simulink model "rotation"  (Simulink 7.0)
settings: Solver=ode45  SolverMode=SingleTasking  StartTime=0.0  StopTime=inf  RelTol=1e-3
values from neighbouring files (symbols this model uses):
  blk = 10    [rotation_init.m]
  col_delx_ws = ceil(col_delx*2^20)    [rotation_init.m]
  col_dely_ws = ceil(col_dely*2^20)    [rotation_init.m]
  fps = 1/(rows*(cols+3*blk))    [rotation_init.m]
  row_delx_ws = ceil(row_delx*2^20)*2    [rotation_init.m]
  row_dely_ws = ceil(row_dely*2^20)*2    [rotation_init.m]
  xstart_init_ws = ceil(xstart_init*2^20)    [rotation_init.m]
  ystart_init_ws = ceil(ystart_init*2^20)    [rotation_init.m]
undefined symbols (not defined in the file or in its folder): cols, rows
libraries: xbsIndex_r4 x273, dspsrcs4 x2, dspsigops x1, vipsrcs x1
(part 1 of 2)
settings Model: Creator=Neelamegam Subramani  LastModifiedBy=IC011758
settings DataIOCC: SaveOutput=off  SignalLogging=off  SaveTime=off

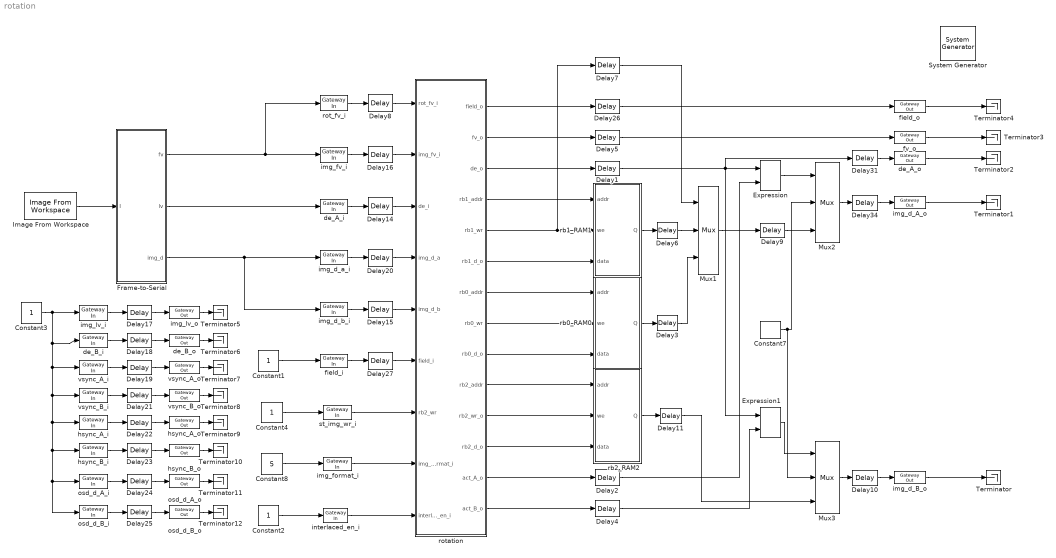
== system rotation ==
  " System Generator" : xbsIndex_r4/ System Generator  Tag=genX  SystemSampleTime=-1  xilinxfamily=spartan3adsp  part=xc3sd3400a  speed=-5  package=fg676  synthesis_tool=XST  clock_wrapper=Clock Enables  directory=./ngc_netlist  testbench=off  simulink_period=(1/fps)/ (rows*(cols+2*blk))  sysclk_period=(1/110e6)*1e9  dcm_input_clock_period=100  incr_netlist=off  trim_vbits=Everywhere in SubSystem  dbl_ovrd=According to Block Masks  core_generation=According to Block Masks  run_coregen=off  deprecated_control=off  eval_field=0  block_type=sysgen
      settings: block_version=8.2
  Constant{1..4} (4 alike) : Constant  OutDataType=sfix(16)  OutScaling=2^0
  Constant7 : xbsIndex_r4/Constant  arith_type=Unsigned  const=0  n_bits=10  bin_pt=0  explicit_period=on  period=(1/fps)/ (rows*(cols+2*blk))  equ=P=C  opselect=C  inp2=PCIN>>17  opr=+  inp1=P  carry=CIN  dbl_ovrd=off  block_type=constant
  Constant8 : Constant  Value=5  OutDataType=sfix(16)  OutScaling=2^0
  Delay1 : xbsIndex_r4/Delay  en=off  latency=5  dbl_ovrd=off  reg_retiming=off  block_type=delay
  Delay{3,6,8..10,14..16,20,27,31,34} (12 alike) : xbsIndex_r4/Delay  en=off  latency=1  dbl_ovrd=off  reg_retiming=off  block_type=delay
      Delay10 settings: infoedit="Delay line having  configurable length.<P><P>Hardware notes: A delay line is a chain, each link of which is an SRL16 followed by a flip-flop. If register retiming is enabled, the delay line is a chain of flip-flops."  xl_area=[0, 0, 0, 0, 0, 0, 0]  block_version=VER_STRING_GOES_HERE
      Delay3 settings: infoedit="Delay line having  configurable length.<P><P>Hardware notes: A delay line is a chain, each link of which is an SRL16 followed by a flip-flop. If register retiming is enabled, the delay line is a chain of flip-flops."  xl_area=[0, 0, 0, 0, 0, 0, 0]  block_version=VER_STRING_GOES_HERE
      Delay31 settings: infoedit="Delay line having  configurable length.<P><P>Hardware notes: A delay line is a chain, each link of which is an SRL16 followed by a flip-flop. If register retiming is enabled, the delay line is a chain of flip-flops."  xl_area=[0, 0, 0, 0, 0, 0, 0]  block_version=VER_STRING_GOES_HERE
      Delay34 settings: infoedit="Delay line having  configurable length.<P><P>Hardware notes: A delay line is a chain, each link of which is an SRL16 followed by a flip-flop. If register retiming is enabled, the delay line is a chain of flip-flops."  xl_area=[0, 0, 0, 0, 0, 0, 0]  block_version=VER_STRING_GOES_HERE
      Delay6 settings: infoedit="Delay line having  configurable length.<P><P>Hardware notes: A delay line is a chain, each link of which is an SRL16 followed by a flip-flop. If register retiming is enabled, the delay line is a chain of flip-flops."  xl_area=[0, 0, 0, 0, 0, 0, 0]  block_version=VER_STRING_GOES_HERE
  Delay11 : xbsIndex_r4/Delay  en=off  latency=2  dbl_ovrd=off  reg_retiming=off  block_type=delay
      settings: infoedit="Delay line having  configurable length.<P><P>Hardware notes: A delay line is a chain, each link of which is an SRL16 followed by a flip-flop. If register retiming is enabled, the delay line is a chain of flip-flops."  xl_area=[0, 0, 0, 0, 0, 0, 0]  block_version=VER_STRING_GOES_HERE
  Delay{17..19,21..25} (8 alike) : xbsIndex_r4/Delay  en=off  latency=15  dbl_ovrd=off  reg_retiming=off  block_type=delay
  Delay2 : xbsIndex_r4/Delay  en=off  latency=5  dbl_ovrd=off  reg_retiming=off  block_type=delay
      settings: infoedit="Delay line having  configurable length.<P><P>Hardware notes: A delay line is a chain, each link of which is an SRL16 followed by a flip-flop. If register retiming is enabled, the delay line is a chain of flip-flops."  xl_area=[0, 0, 0, 0, 0, 0, 0]  block_version=VER_STRING_GOES_HERE
  Delay26 : xbsIndex_r4/Delay  en=off  latency=6  dbl_ovrd=off  reg_retiming=off  block_type=delay
  Delay4 : xbsIndex_r4/Delay  en=off  latency=5  dbl_ovrd=off  reg_retiming=off  block_type=delay
      settings: infoedit="Delay line having  configurable length.<P><P>Hardware notes: A delay line is a chain, each link of which is an SRL16 followed by a flip-flop. If register retiming is enabled, the delay line is a chain of flip-flops."  xl_area=[0, 0, 0, 0, 0, 0, 0]  block_version=VER_STRING_GOES_HERE
  Delay5 : xbsIndex_r4/Delay  en=off  latency=6  dbl_ovrd=off  reg_retiming=off  block_type=delay
  Delay7 : xbsIndex_r4/Delay  en=off  latency=3  dbl_ovrd=off  reg_retiming=off  block_type=delay
      settings: infoedit="Delay line having  configurable length.<P><P>Hardware notes: A delay line is a chain, each link of which is an SRL16 followed by a flip-flop. If register retiming is enabled, the delay line is a chain of flip-flops."  xl_area=[0, 0, 0, 0, 0, 0, 0]  block_version=VER_STRING_GOES_HERE
  Expression : xbsIndex_r4/Expression  expression=a & b  align_bp=on  en=off  latency=0  precision=Full  arith_type=Unsigned  n_bits=16  bin_pt=0  dbl_ovrd=off  block_type=expr
      settings: block_version=10.1.3
  Expression1 : xbsIndex_r4/Expression  expression=a & b  align_bp=on  en=off  latency=0  precision=Full  arith_type=Unsigned  n_bits=16  bin_pt=0  dbl_ovrd=off  block_type=expr
      settings: block_version=10.1.3
  Frame-to-Serial : Subsystem
  Image From Workspace : vipsrcs/Image From Workspace  Tag=vipblks_nd  SystemSampleTime=-1  ImageValue=in  Ts=1/fps  imagePorts=One multidimensional signal  ImageDataType=double  Signed=on  WordLength=16  sdImageDataType=sfix(16)  FractionLengthMode=User-defined  FractionLength=15  OutPortLabels=R|G|B
      link override Constant1: Value=ImageValue
  Mux1 : xbsIndex_r4/Mux  inputs=2  en=off  latency=0  precision=Full  arith_type=Unsigned  n_bits=16  bin_pt=14  quantization=Truncate  overflow=Wrap  dbl_ovrd=off  block_type=mux
  Mux2 : xbsIndex_r4/Mux  inputs=2  en=off  latency=0  precision=Full  arith_type=Unsigned  n_bits=16  bin_pt=14  quantization=Truncate  overflow=Wrap  dbl_ovrd=off  block_type=mux
  Mux3 : xbsIndex_r4/Mux  inputs=2  en=off  latency=0  precision=Full  arith_type=Unsigned  n_bits=16  bin_pt=14  quantization=Truncate  overflow=Wrap  dbl_ovrd=off  block_type=mux
  Terminator{,1..12} (13 alike) : Terminator
  de_A_i : xbsIndex_r4/Gateway In  arith_type=Boolean  n_bits=10  bin_pt=0  quantization=Truncate  overflow=Wrap  period=(1/fps)/ (rows*(cols+2*blk))  dbl_ovrd=off  timing_constraint=None  locs_specified=off  LOCs={}  block_type=gatewayin
      settings: infoedit="Gateway in block.  Converts inputs of type Simulink integer, double and fixed point to  Xilinx fixed point type.<P><P>Hardware notes:  In hardware these blocks become top level input ports."  block_version=10.1.3
  de_A_o : xbsIndex_r4/Gateway Out  hdl_port=on  timing_constraint=None  locs_specified=off  LOCs={'AC11'}  block_type=gatewayout
      settings: infoedit="Gateway out block.  Converts Xilinx fixed point inputs into ouputs of type Simulink integer, double, or fixed point.<P><P>Hardware notes:  In hardware these blocks become top level output ports or are discarded, depending on how they are configured."  block_version=10.1.3
  de_B_i : xbsIndex_r4/Gateway In  arith_type=Boolean  n_bits=10  bin_pt=0  quantization=Truncate  overflow=Wrap  period=(1/fps)/ (rows*(cols+2*blk))  dbl_ovrd=off  timing_constraint=None  locs_specified=off  LOCs={}  block_type=gatewayin
      settings: infoedit="Gateway in block.  Converts inputs of type Simulink integer, double and fixed point to  Xilinx fixed point type.<P><P>Hardware notes:  In hardware these blocks become top level input ports."  block_version=10.1.3
  de_B_o : xbsIndex_r4/Gateway Out  hdl_port=on  timing_constraint=None  locs_specified=off  LOCs={}  block_type=gatewayout
      settings: infoedit="Gateway out block.  Converts Xilinx fixed point inputs into ouputs of type Simulink integer, double, or fixed point.<P><P>Hardware notes:  In hardware these blocks become top level output ports or are discarded, depending on how they are configured."  block_version=10.1.3
  field_i : xbsIndex_r4/Gateway In  arith_type=Boolean  n_bits=16  bin_pt=14  quantization="Round  (unbiased: +/- Inf)"  overflow=Saturate  period=(1/fps)/ (rows*(cols+2*blk))  dbl_ovrd=off  timing_constraint=None  locs_specified=off  LOCs={}  block_type=gatewayin
      settings: infoedit="Gateway in block.  Converts inputs of type Simulink integer, double and fixed point to  Xilinx fixed point type.<P><P>Hardware notes:  In hardware these blocks become top level input ports."  block_version=10.1.3
  field_o : xbsIndex_r4/Gateway Out  hdl_port=on  timing_constraint=None  locs_specified=off  LOCs={}  block_type=gatewayout
      settings: infoedit="Gateway out block.  Converts Xilinx fixed point inputs into ouputs of type Simulink integer, double, or fixed point.<P><P>Hardware notes:  In hardware these blocks become top level output ports or are discarded, depending on how they are configured."  block_version=10.1.3
  fv_o : xbsIndex_r4/Gateway Out  hdl_port=on  timing_constraint=None  locs_specified=off  LOCs={'AD11'}  block_type=gatewayout
      settings: infoedit="Gateway out block.  Converts Xilinx fixed point inputs into ouputs of type Simulink integer, double, or fixed point.<P><P>Hardware notes:  In hardware these blocks become top level output ports or are discarded, depending on how they are configured."  block_version=10.1.3
  hsync_A_i : xbsIndex_r4/Gateway In  arith_type=Boolean  n_bits=10  bin_pt=0  quantization=Truncate  overflow=Wrap  period=(1/fps)/ (rows*(cols+2*blk))  dbl_ovrd=off  timing_constraint=None  locs_specified=off  LOCs={}  block_type=gatewayin
      settings: infoedit="Gateway in block.  Converts inputs of type Simulink integer, double and fixed point to  Xilinx fixed point type.<P><P>Hardware notes:  In hardware these blocks become top level input ports."  block_version=10.1.3
  hsync_A_o : xbsIndex_r4/Gateway Out  hdl_port=on  timing_constraint=None  locs_specified=off  LOCs={}  block_type=gatewayout
      settings: infoedit="Gateway out block.  Converts Xilinx fixed point inputs into ouputs of type Simulink integer, double, or fixed point.<P><P>Hardware notes:  In hardware these blocks become top level output ports or are discarded, depending on how they are configured."  block_version=10.1.3
  hsync_B_i : xbsIndex_r4/Gateway In  arith_type=Boolean  n_bits=10  bin_pt=0  quantization=Truncate  overflow=Wrap  period=(1/fps)/ (rows*(cols+2*blk))  dbl_ovrd=off  timing_constraint=None  locs_specified=off  LOCs={}  block_type=gatewayin
      settings: infoedit="Gateway in block.  Converts inputs of type Simulink integer, double and fixed point to  Xilinx fixed point type.<P><P>Hardware notes:  In hardware these blocks become top level input ports."  block_version=10.1.3
  hsync_B_o : xbsIndex_r4/Gateway Out  hdl_port=on  timing_constraint=None  locs_specified=off  LOCs={}  block_type=gatewayout
      settings: infoedit="Gateway out block.  Converts Xilinx fixed point inputs into ouputs of type Simulink integer, double, or fixed point.<P><P>Hardware notes:  In hardware these blocks become top level output ports or are discarded, depending on how they are configured."  block_version=10.1.3
  img_d_A_o : xbsIndex_r4/Gateway Out  hdl_port=on  timing_constraint=None  locs_specified=off  LOCs={}  block_type=gatewayout
      settings: infoedit="Gateway out block.  Converts Xilinx fixed point inputs into ouputs of type Simulink integer, double, or fixed point.<P><P>Hardware notes:  In hardware these blocks become top level output ports or are discarded, depending on how they are configured."  block_version=10.1.3
  img_d_B_o : xbsIndex_r4/Gateway Out  hdl_port=on  timing_constraint=None  locs_specified=off  LOCs={}  block_type=gatewayout
      settings: infoedit="Gateway out block.  Converts Xilinx fixed point inputs into ouputs of type Simulink integer, double, or fixed point.<P><P>Hardware notes:  In hardware these blocks become top level output ports or are discarded, depending on how they are configured."  block_version=10.1.3
  img_d_a_i : xbsIndex_r4/Gateway In  arith_type=Unsigned  n_bits=10  bin_pt=0  quantization=Truncate  overflow=Wrap  period=(1/fps)/ (rows*(cols+2*blk))  dbl_ovrd=off  timing_constraint=None  locs_specified=off  LOCs={}  block_type=gatewayin
      settings: infoedit="Gateway in block.  Converts inputs of type Simulink integer, double and fixed point to  Xilinx fixed point type.<P><P>Hardware notes:  In hardware these blocks become top level input ports."  block_version=10.1.3
  img_d_b_i : xbsIndex_r4/Gateway In  arith_type=Unsigned  n_bits=10  bin_pt=0  quantization=Truncate  overflow=Wrap  period=(1/fps)/ (rows*(cols+2*blk))  dbl_ovrd=off  timing_constraint=None  locs_specified=off  LOCs={}  block_type=gatewayin
      settings: infoedit="Gateway in block.  Converts inputs of type Simulink integer, double and fixed point to  Xilinx fixed point type.<P><P>Hardware notes:  In hardware these blocks become top level input ports."  block_version=10.1.3
  img_format_i : xbsIndex_r4/Gateway In  arith_type=Unsigned  n_bits=3  bin_pt=0  quantization=Truncate  overflow=Wrap  period=(1/fps)/ (rows*(cols+2*blk))  dbl_ovrd=off  timing_constraint=None  locs_specified=off  LOCs={}  block_type=gatewayin
      settings: infoedit="Gateway in block.  Converts inputs of type Simulink integer, double and fixed point to  Xilinx fixed point type.<P><P>Hardware notes:  In hardware these blocks become top level input ports."  block_version=10.1.3
  img_fv_i : xbsIndex_r4/Gateway In  arith_type=Boolean  n_bits=16  bin_pt=14  quantization="Round  (unbiased: +/- Inf)"  overflow=Saturate  period=(1/fps)/ (rows*(cols+2*blk))  dbl_ovrd=off  timing_constraint=None  locs_specified=off  LOCs={}  block_type=gatewayin
      settings: infoedit="Gateway in block.  Converts inputs of type Simulink integer, double and fixed point to  Xilinx fixed point type.<P><P>Hardware notes:  In hardware these blocks become top level input ports."  block_version=10.1.3
  img_lv_i : xbsIndex_r4/Gateway In  arith_type=Boolean  n_bits=16  bin_pt=14  quantization="Round  (unbiased: +/- Inf)"  overflow=Saturate  period=(1/fps)/ (rows*(cols+2*blk))  dbl_ovrd=off  timing_constraint=None  locs_specified=off  LOCs={}  block_type=gatewayin
      settings: infoedit="Gateway in block.  Converts inputs of type Simulink integer, double and fixed point to  Xilinx fixed point type.<P><P>Hardware notes:  In hardware these blocks become top level input ports."  block_version=10.1.3
  img_lv_o : xbsIndex_r4/Gateway Out  hdl_port=on  timing_constraint=None  locs_specified=off  LOCs={}  block_type=gatewayout
      settings: infoedit="Gateway out block.  Converts Xilinx fixed point inputs into ouputs of type Simulink integer, double, or fixed point.<P><P>Hardware notes:  In hardware these blocks become top level output ports or are discarded, depending on how they are configured."  block_version=10.1.3
  interlaced_en_i : xbsIndex_r4/Gateway In  arith_type=Boolean  n_bits=16  bin_pt=14  quantization="Round  (unbiased: +/- Inf)"  overflow=Saturate  period=(1/fps)/ (rows*(cols+2*blk))  dbl_ovrd=off  timing_constraint=None  locs_specified=off  LOCs={}  block_type=gatewayin
      settings: infoedit="Gateway in block.  Converts inputs of type Simulink integer, double and fixed point to  Xilinx fixed point type.<P><P>Hardware notes:  In hardware these blocks become top level input ports."  block_version=10.1.3
  osd_d_A_i : xbsIndex_r4/Gateway In  arith_type=Unsigned  n_bits=2  bin_pt=0  quantization=Truncate  overflow=Wrap  period=(1/fps)/ (rows*(cols+2*blk))  dbl_ovrd=off  timing_constraint=None  locs_specified=off  LOCs={}  block_type=gatewayin
      settings: infoedit="Gateway in block.  Converts inputs of type Simulink integer, double and fixed point to  Xilinx fixed point type.<P><P>Hardware notes:  In hardware these blocks become top level input ports."  block_version=10.1.3
  osd_d_A_o : xbsIndex_r4/Gateway Out  hdl_port=on  timing_constraint=None  locs_specified=off  LOCs={}  block_type=gatewayout
      settings: infoedit="Gateway out block.  Converts Xilinx fixed point inputs into ouputs of type Simulink integer, double, or fixed point.<P><P>Hardware notes:  In hardware these blocks become top level output ports or are discarded, depending on how they are configured."  block_version=10.1.3
  osd_d_B_i : xbsIndex_r4/Gateway In  arith_type=Unsigned  n_bits=2  bin_pt=0  quantization=Truncate  overflow=Wrap  period=(1/fps)/ (rows*(cols+2*blk))  dbl_ovrd=off  timing_constraint=None  locs_specified=off  LOCs={}  block_type=gatewayin
      settings: infoedit="Gateway in block.  Converts inputs of type Simulink integer, double and fixed point to  Xilinx fixed point type.<P><P>Hardware notes:  In hardware these blocks become top level input ports."  block_version=10.1.3
  osd_d_B_o : xbsIndex_r4/Gateway Out  hdl_port=on  timing_constraint=None  locs_specified=off  LOCs={}  block_type=gatewayout
      settings: infoedit="Gateway out block.  Converts Xilinx fixed point inputs into ouputs of type Simulink integer, double, or fixed point.<P><P>Hardware notes:  In hardware these blocks become top level output ports or are discarded, depending on how they are configured."  block_version=10.1.3
  rb0_RAM0 : Subsystem  AncestorBlock=XtremeDSPKit_r4/External RAM  mask(XtremeDSP Kit External Memory){zbt_data_read_arith_type=Unsigned, zbt_data_width=16, zbt_data_bin_pt=0}
      mask prompts: zbt_data_read_arith_type "Output Data Type"; zbt_data_width "Data Width"; zbt_data_bin_pt "Data Binary Point (from 0 to 16)"
      mask help: 256K x 16 External Memory
      mask init:
      | i = imread('xtreme.jpg');
      mask Help: eval('');xlDoc('-book','sysgen','-topic','XtremeDSP_External_RAM');
      mask StyleString: popup(Unsigned|Signed  (2's comp)),edit,edit
      mask Display:
      | image(i);
      | port_label ('input', 1, 'addr');
      | port_label ('input', 2, 'we');
      | port_label ('input', 3, 'data');
  rb1_RAM1 : Subsystem  AncestorBlock=XtremeDSPKit_r4/External RAM  mask(XtremeDSP Kit External Memory){zbt_data_read_arith_type=Unsigned, zbt_data_width=16, zbt_data_bin_pt=0}
      mask prompts: zbt_data_read_arith_type "Output Data Type"; zbt_data_width "Data Width"; zbt_data_bin_pt "Data Binary Point (from 0 to 16)"
      mask help: 256K x 16 External Memory
      mask init:
      | i = imread('xtreme.jpg');
      mask Help: eval('');xlDoc('-book','sysgen','-topic','XtremeDSP_External_RAM');
      mask StyleString: popup(Unsigned|Signed  (2's comp)),edit,edit
      mask Display:
      | image(i);
      | port_label ('input', 1, 'addr');
      | port_label ('input', 2, 'we');
      | port_label ('input', 3, 'data');
  rb2_RAM2 : Subsystem  AncestorBlock=XtremeDSPKit_r4/External RAM  mask(XtremeDSP Kit External Memory){zbt_data_read_arith_type=Unsigned, zbt_data_width=16, zbt_data_bin_pt=0}
      mask prompts: zbt_data_read_arith_type "Output Data Type"; zbt_data_width "Data Width"; zbt_data_bin_pt "Data Binary Point (from 0 to 16)"
      mask help: 256K x 16 External Memory
      mask init:
      | i = imread('xtreme.jpg');
      mask Help: eval('');xlDoc('-book','sysgen','-topic','XtremeDSP_External_RAM');
      mask StyleString: popup(Unsigned|Signed  (2's comp)),edit,edit
      mask Display:
      | image(i);
      | port_label ('input', 1, 'addr');
      | port_label ('input', 2, 'we');
      | port_label ('input', 3, 'data');
  rot_fv_i : xbsIndex_r4/Gateway In  arith_type=Boolean  n_bits=16  bin_pt=14  quantization="Round  (unbiased: +/- Inf)"  overflow=Saturate  period=(1/fps)/ (rows*(cols+2*blk))  dbl_ovrd=off  timing_constraint=None  locs_specified=off  LOCs={}  block_type=gatewayin
      settings: infoedit="Gateway in block.  Converts inputs of type Simulink integer, double and fixed point to  Xilinx fixed point type.<P><P>Hardware notes:  In hardware these blocks become top level input ports."  block_version=10.1.3
  rotation : Subsystem
  st_img_wr_i : xbsIndex_r4/Gateway In  arith_type=Boolean  n_bits=10  bin_pt=0  quantization=Truncate  overflow=Wrap  period=(1/fps)/ (rows*(cols+2*blk))  dbl_ovrd=off  timing_constraint=None  locs_specified=off  LOCs={}  block_type=gatewayin
      settings: infoedit="Gateway in block.  Converts inputs of type Simulink integer, double and fixed point to  Xilinx fixed point type.<P><P>Hardware notes:  In hardware these blocks become top level input ports."  block_version=10.1.3
  vsync_A_i : xbsIndex_r4/Gateway In  arith_type=Boolean  n_bits=10  bin_pt=0  quantization=Truncate  overflow=Wrap  period=(1/fps)/ (rows*(cols+2*blk))  dbl_ovrd=off  timing_constraint=None  locs_specified=off  LOCs={}  block_type=gatewayin
      settings: infoedit="Gateway in block.  Converts inputs of type Simulink integer, double and fixed point to  Xilinx fixed point type.<P><P>Hardware notes:  In hardware these blocks become top level input ports."  block_version=10.1.3
  vsync_A_o : xbsIndex_r4/Gateway Out  hdl_port=on  timing_constraint=None  locs_specified=off  LOCs={}  block_type=gatewayout
      settings: infoedit="Gateway out block.  Converts Xilinx fixed point inputs into ouputs of type Simulink integer, double, or fixed point.<P><P>Hardware notes:  In hardware these blocks become top level output ports or are discarded, depending on how they are configured."  block_version=10.1.3
  vsync_B_i : xbsIndex_r4/Gateway In  arith_type=Boolean  n_bits=10  bin_pt=0  quantization=Truncate  overflow=Wrap  period=(1/fps)/ (rows*(cols+2*blk))  dbl_ovrd=off  timing_constraint=None  locs_specified=off  LOCs={}  block_type=gatewayin
      settings: infoedit="Gateway in block.  Converts inputs of type Simulink integer, double and fixed point to  Xilinx fixed point type.<P><P>Hardware notes:  In hardware these blocks become top level input ports."  block_version=10.1.3
  vsync_B_o : xbsIndex_r4/Gateway Out  hdl_port=on  timing_constraint=None  locs_specified=off  LOCs={}  block_type=gatewayout
      settings: infoedit="Gateway out block.  Converts Xilinx fixed point inputs into ouputs of type Simulink integer, double, or fixed point.<P><P>Hardware notes:  In hardware these blocks become top level output ports or are discarded, depending on how they are configured."  block_version=10.1.3
  wires:
  Image From Workspace/1 -> Frame-to-Serial/1(I)
  rb1_RAM1/1(Q) -> Delay6/1
  rb0_RAM0/1(Q) -> Delay3/1
  Delay6/1 -> Mux1/2
  Delay3/1 -> Mux1/3
  Delay7/1 -> Mux1/1
  Mux1/1 -> Delay9/1
  rb2_RAM2/1(Q) -> Delay11/1
  img_d_B_o/1 -> Terminator/1
  img_d_a_i/1 -> Delay20/1
  Frame-to-Serial/2(lv) -> de_A_i/1
  Frame-to-Serial/3(img_d) -> img_d_a_i/1, img_d_b_i/1
  de_A_i/1 -> Delay14/1
  img_fv_i/1 -> Delay16/1
  Constant1/1 -> field_i/1
  img_d_b_i/1 -> Delay15/1
  field_i/1 -> Delay27/1
  Delay17/1 -> img_lv_o/1
  de_B_i/1 -> Delay18/1
  Delay18/1 -> de_B_o/1
  vsync_A_i/1 -> Delay19/1
  Delay19/1 -> vsync_A_o/1
  vsync_B_i/1 -> Delay21/1
  Delay21/1 -> vsync_B_o/1
  hsync_A_i/1 -> Delay22/1
  Delay22/1 -> hsync_A_o/1
  hsync_B_i/1 -> Delay23/1
  Delay23/1 -> hsync_B_o/1
  osd_d_A_i/1 -> Delay24/1
  Delay24/1 -> osd_d_A_o/1
  osd_d_B_i/1 -> Delay25/1
  Delay25/1 -> osd_d_B_o/1
  Constant3/1 -> osd_d_B_i/1, osd_d_A_i/1, hsync_B_i/1, hsync_A_i/1, vsync_B_i/1, vsync_A_i/1, de_B_i/1, img_lv_i/1
  img_lv_i/1 -> Delay17/1
  Frame-to-Serial/1(fv) -> img_fv_i/1, rot_fv_i/1
  rotation/12(rb2_d_o) -> rb2_RAM2/3(data)
  rotation/11(rb2_wr_o) -> rb2_RAM2/2(we)
  rotation/10(rb2_addr) -> rb2_RAM2/1(addr)
  rotation/9(rb0_d_o) -> rb0_RAM0/3(data)
  rotation/8(rb0_wr) -> rb0_RAM0/2(we)
  rotation/7(rb0_addr) -> rb0_RAM0/1(addr)
  rotation/6(rb1_d_o) -> rb1_RAM1/3(data)
  rotation/5(rb1_wr) -> Delay7/1, rb1_RAM1/2(we)
  rotation/4(rb1_addr) -> rb1_RAM1/1(addr)
  img_d_A_o/1 -> Terminator1/1
  Delay14/1 -> rotation/3(de_i)
  Delay20/1 -> rotation/4(img_d_a)
  Delay15/1 -> rotation/5(img_d_b)
  Delay27/1 -> rotation/6(field_i)
  Constant4/1 -> st_img_wr_i/1
  rotation/1(field_o) -> Delay26/1
  de_A_o/1 -> Terminator2/1
  fv_o/1 -> Terminator3/1
  field_o/1 -> Terminator4/1
  img_lv_o/1 -> Terminator5/1
  de_B_o/1 -> Terminator6/1
  vsync_A_o/1 -> Terminator7/1
  vsync_B_o/1 -> Terminator8/1
  hsync_A_o/1 -> Terminator9/1
  hsync_B_o/1 -> Terminator10/1
  osd_d_A_o/1 -> Terminator11/1
  osd_d_B_o/1 -> Terminator12/1
  Delay9/1 -> Mux2/3
  Mux2/1 -> Delay34/1
  Constant7/1 -> Mux2/2, Mux3/2
  Delay31/1 -> de_A_o/1
  Delay34/1 -> img_d_A_o/1
  img_format_i/1 -> rotation/8(img_format_i)
  Constant8/1 -> img_format_i/1
  Delay1/1 -> Delay31/1, Expression/1, Expression1/1
  rotation/3(de_o) -> Delay1/1
  Delay5/1 -> fv_o/1
  rotation/2(fv_o) -> Delay5/1
  Delay26/1 -> field_o/1
  st_img_wr_i/1 -> rotation/7(rb2_wr)
  rotation/13(act_A_o) -> Delay2/1
  rotation/14(act_B_o) -> Delay4/1
  Delay2/1 -> Expression/2
  Expression/1 -> Mux2/1
  Delay4/1 -> Expression1/2
  Expression1/1 -> Mux3/1
  Delay11/1 -> Mux3/3
  Mux3/1 -> Delay10/1
  Delay10/1 -> img_d_B_o/1
  rot_fv_i/1 -> Delay8/1
  Delay8/1 -> rotation/1(rot_fv_i)
  Delay16/1 -> rotation/2(img_fv_i)
  Constant2/1 -> interlaced_en_i/1
  interlaced_en_i/1 -> rotation/9(interlaced_en_i)

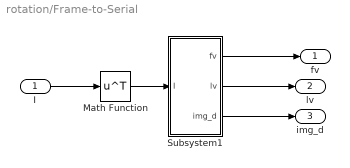
== system rotation/Frame-to-Serial ==
  I : Inport  OutDataType=sfix(16)  OutScaling=2^0
  Math Function : Math  Operator=transpose  SampleTime=(1/fps)  OutDataType=sfix(16)  OutScaling=2^0  SaturateOnIntegerOverflow=on
  Subsystem1 : Subsystem
  fv : Outport  OutDataType=sfix(16)  OutScaling=2^0
  lv : Outport  Port=2  OutDataType=sfix(16)  OutScaling=2^0
  img_d : Outport  Port=3  OutDataType=sfix(16)  OutScaling=2^0
  wires:
  I/1 -> Math Function/1
  Math Function/1 -> Subsystem1/1(I)
  Subsystem1/1(fv) -> fv/1
  Subsystem1/2(lv) -> lv/1
  Subsystem1/3(img_d) -> img_d/1

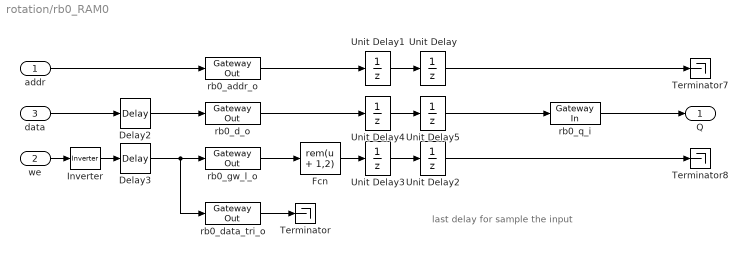
== system rotation/rb0_RAM0 ==
  note: last delay for sample the input
  addr : Inport  OutDataType=sfix(16)  OutScaling=2^0
  we : Inport  Port=2  OutDataType=sfix(16)  OutScaling=2^0
  data : Inport  Port=3  OutDataType=sfix(16)  OutScaling=2^0
  Delay2 : xbsIndex_r4/Delay  en=off  latency=1  dbl_ovrd=off  reg_retiming=off  block_type=delay
      settings: infoedit="Delay line having  configurable length.<P><P>Hardware notes: A delay line is a chain, each link of which is an SRL16 followed by a flip-flop. If register retiming is enabled, the delay line is a chain of flip-flops."  xl_area=[0, 0, 0, 0, 0, 0, 0]  block_version=VER_STRING_GOES_HERE
  Delay3 : xbsIndex_r4/Delay  en=off  latency=1  dbl_ovrd=off  reg_retiming=off  block_type=delay
      settings: infoedit="Delay line having  configurable length.<P><P>Hardware notes: A delay line is a chain, each link of which is an SRL16 followed by a flip-flop. If register retiming is enabled, the delay line is a chain of flip-flops."  xl_area=[0, 0, 0, 0, 0, 0, 0]  block_version=VER_STRING_GOES_HERE
  Fcn : Fcn  Expr=rem(u + 1,2)  SampleTime=(1/fps)/ (rows*(cols+2*blk))
  Inverter : xbsIndex_r4/Inverter  en=off  latency=0  dbl_ovrd=off  block_type=inv
      settings: xl_area=[0, 0, 0, 0, 0, 0, 0]  block_version=VER_STRING_GOES_HERE
  Terminator : Terminator
  Terminator7 : Terminator
  Terminator8 : Terminator
  Unit Delay{,1..5} (6 alike) : UnitDelay  SampleTime=(1/fps)/ (rows*(cols+2*blk))
  rb0_addr_o : xbsIndex_r4/Gateway Out  hdl_port=on  timing_constraint="Data Rate;  Set 'FAST' Attribute"  locs_specified=off  LOCs={'U1','U2','K6','L7','M10','M9','V2','V1','U4','T5','K3','K2','J5','J4','K5','K4','L4','L3'}  block_type=gatewayout
      settings: infoedit="Gateway out block.  Converts Xilinx fixed point inputs into ouputs of type Simulink integer, double, or fixed point.<P><P>Hardware notes:  In hardware these blocks become top level output ports or are discarded, depending on how they are configured."  xl_area=[0, 0, 0, 0, 0, 0, 0]  sginterface={'Nallatech'=>{'xdspkit'=>{'non_memory_mapped_port'=>'zbt_addr'}},'Xilinx'=>{'jtaghwcosim'=>{'non_memory_mapped_port'=>'zbt_addr'},'xdspkit'=>{'non_memory_mapped_port'=>'zbt_addr'}}}  block_version=VER_STRING_GOES_HERE
  rb0_d_o : xbsIndex_r4/Gateway Out  hdl_port=on  timing_constraint=None  locs_specified=off  LOCs={'B21','B22','A22','B23','B19','C19','A20','A21','A23','B24','A24','A25','E18','D18','C18','B18'}  block_type=gatewayout
      settings: infoedit="Gateway out block.  Converts Xilinx fixed point inputs into ouputs of type Simulink integer, double, or fixed point.<P><P>Hardware notes:  In hardware these blocks become top level output ports or are discarded, depending on how they are configured."  xl_area=[0, 0, 0, 0, 0, 0, 0]  sginterface={'Nallatech'=>{'xdspkit'=>{'non_memory_mapped_port'=>'zbt_data'}},'Xilinx'=>{'jtaghwcosim'=>{'non_memory_mapped_port'=>'zbt_data'},'xdspkit'=>{'non_memory_mapped_port'=>'zbt_data'}}}  block_version=VER_STRING_GOES_HERE
  rb0_data_tri_o : xbsIndex_r4/Gateway Out  hdl_port=on  timing_constraint=None  locs_specified=off  LOCs={}  block_type=gatewayout
      settings: infoedit="Gateway out block.  Converts Xilinx fixed point inputs into ouputs of type Simulink integer, double, or fixed point.<P><P>Hardware notes:  In hardware these blocks become top level output ports or are discarded, depending on how they are configured."  xl_area=[0, 0, 0, 0, 0, 0, 0]  sginterface={'Nallatech'=>{'xdspkit'=>{'non_memory_mapped_port'=>'zbt_data_tri'}},'Xilinx'=>{'jtaghwcosim'=>{'non_memory_mapped_port'=>'zbt_data_tri'},'xdspkit'=>{'non_memory_mapped_port'=>'zbt_data_tri'}}}  block_version=VER_STRING_GOES_HERE
  rb0_gw_l_o : xbsIndex_r4/Gateway Out  hdl_port=on  timing_constraint=None  locs_specified=off  LOCs={'A14'}  block_type=gatewayout
      settings: infoedit="Gateway out block.  Converts Xilinx fixed point inputs into ouputs of type Simulink integer, double, or fixed point.<P><P>Hardware notes:  In hardware these blocks become top level output ports or are discarded, depending on how they are configured."  xl_area=[0, 0, 0, 0, 0, 0, 0]  sginterface={'Nallatech'=>{'xdspkit'=>{'non_memory_mapped_port'=>'zbt_rd_wr'}},'Xilinx'=>{'jtaghwcosim'=>{'non_memory_mapped_port'=>'zbt_rd_wr'},'xdspkit'=>{'non_memory_mapped_port'=>'zbt_rd_wr'}}}  block_version=VER_STRING_GOES_HERE
  rb0_q_i : xbsIndex_r4/Gateway In  arith_type=Unsigned  n_bits=10  bin_pt=0  quantization=Truncate  overflow=Wrap  period=(1/fps)/ (rows*(cols+2*blk))  dbl_ovrd=off  timing_constraint=None  locs_specified=off  LOCs={}  block_type=gatewayin
      settings: infoedit="Gateway in block.  Converts inputs of type Simulink integer, double and fixed point to  Xilinx fixed point type.<P><P>Hardware notes:  In hardware these blocks become top level input ports."  xl_area=[0, 0, 0, 0, 0, 0, 0]  sginterface={'Nallatech'=>{'xdspkit'=>{'non_memory_mapped_port'=>'zbt_data_read'}},'Xilinx'=>{'jtaghwcosim'=>{'non_memory_mapped_port'=>'zbt_data_read'},'xdspkit'=>{'non_memory_mapped_port'=>'zbt_data_read'}}}  block_version=VER_STRING_GOES_HERE
  Q : Outport  OutDataType=sfix(16)  OutScaling=2^0
  wires:
  Inverter/1 -> Delay3/1
  Fcn/1 -> Unit Delay3/1
  rb0_gw_l_o/1 -> Fcn/1
  data/1 -> Delay2/1
  rb0_data_tri_o/1 -> Terminator/1
  addr/1 -> rb0_addr_o/1
  we/1 -> Inverter/1
  Unit Delay1/1 -> Unit Delay/1
  rb0_addr_o/1 -> Unit Delay1/1
  Unit Delay3/1 -> Unit Delay2/1
  rb0_q_i/1 -> Q/1
  Unit Delay/1 -> Terminator7/1
  rb0_d_o/1 -> Unit Delay4/1
  Unit Delay2/1 -> Terminator8/1
  Delay2/1 -> rb0_d_o/1
  Unit Delay4/1 -> Unit Delay5/1
  Unit Delay5/1 -> rb0_q_i/1
  Delay3/1 -> rb0_gw_l_o/1, rb0_data_tri_o/1

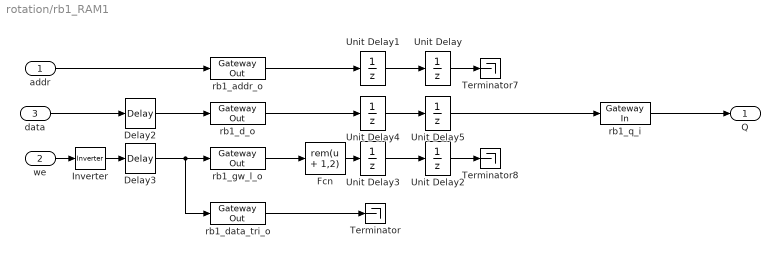
== system rotation/rb1_RAM1 ==
  addr : Inport  OutDataType=sfix(16)  OutScaling=2^0
  we : Inport  Port=2  OutDataType=sfix(16)  OutScaling=2^0
  data : Inport  Port=3  OutDataType=sfix(16)  OutScaling=2^0
  Delay2 : xbsIndex_r4/Delay  en=off  latency=1  dbl_ovrd=off  reg_retiming=off  block_type=delay
      settings: infoedit="Delay line having  configurable length.<P><P>Hardware notes: A delay line is a chain, each link of which is an SRL16 followed by a flip-flop. If register retiming is enabled, the delay line is a chain of flip-flops."  xl_area=[0, 0, 0, 0, 0, 0, 0]  block_version=VER_STRING_GOES_HERE
  Delay3 : xbsIndex_r4/Delay  en=off  latency=1  dbl_ovrd=off  reg_retiming=off  block_type=delay
      settings: infoedit="Delay line having  configurable length.<P><P>Hardware notes: A delay line is a chain, each link of which is an SRL16 followed by a flip-flop. If register retiming is enabled, the delay line is a chain of flip-flops."  xl_area=[0, 0, 0, 0, 0, 0, 0]  block_version=VER_STRING_GOES_HERE
  Fcn : Fcn  Expr=rem(u + 1,2)  SampleTime=(1/fps)/ (rows*(cols+2*blk))
  Inverter : xbsIndex_r4/Inverter  en=off  latency=0  dbl_ovrd=off  block_type=inv
      settings: xl_area=[0, 0, 0, 0, 0, 0, 0]  block_version=VER_STRING_GOES_HERE
  Terminator : Terminator
  Terminator7 : Terminator
  Terminator8 : Terminator
  Unit Delay{,1..5} (6 alike) : UnitDelay  SampleTime=(1/fps)/ (rows*(cols+2*blk))
  rb1_addr_o : xbsIndex_r4/Gateway Out  hdl_port=on  timing_constraint="Data Rate;  Set 'FAST' Attribute"  locs_specified=off  LOCs={'U1','U2','K6','L7','M10','M9','V2','V1','U4','T5','K3','K2','J5','J4','K5','K4','L4','L3'}  block_type=gatewayout
      settings: infoedit="Gateway out block.  Converts Xilinx fixed point inputs into ouputs of type Simulink integer, double, or fixed point.<P><P>Hardware notes:  In hardware these blocks become top level output ports or are discarded, depending on how they are configured."  xl_area=[0, 0, 0, 0, 0, 0, 0]  sginterface={'Nallatech'=>{'xdspkit'=>{'non_memory_mapped_port'=>'zbt_addr'}},'Xilinx'=>{'jtaghwcosim'=>{'non_memory_mapped_port'=>'zbt_addr'},'xdspkit'=>{'non_memory_mapped_port'=>'zbt_addr'}}}  block_version=VER_STRING_GOES_HERE
  rb1_d_o : xbsIndex_r4/Gateway Out  hdl_port=on  timing_constraint=None  locs_specified=off  LOCs={'B21','B22','A22','B23','B19','C19','A20','A21','A23','B24','A24','A25','E18','D18','C18','B18'}  block_type=gatewayout
      settings: infoedit="Gateway out block.  Converts Xilinx fixed point inputs into ouputs of type Simulink integer, double, or fixed point.<P><P>Hardware notes:  In hardware these blocks become top level output ports or are discarded, depending on how they are configured."  xl_area=[0, 0, 0, 0, 0, 0, 0]  sginterface={'Nallatech'=>{'xdspkit'=>{'non_memory_mapped_port'=>'zbt_data'}},'Xilinx'=>{'jtaghwcosim'=>{'non_memory_mapped_port'=>'zbt_data'},'xdspkit'=>{'non_memory_mapped_port'=>'zbt_data'}}}  block_version=VER_STRING_GOES_HERE
  rb1_data_tri_o : xbsIndex_r4/Gateway Out  hdl_port=on  timing_constraint=None  locs_specified=off  LOCs={}  block_type=gatewayout
      settings: infoedit="Gateway out block.  Converts Xilinx fixed point inputs into ouputs of type Simulink integer, double, or fixed point.<P><P>Hardware notes:  In hardware these blocks become top level output ports or are discarded, depending on how they are configured."  xl_area=[0, 0, 0, 0, 0, 0, 0]  sginterface={'Nallatech'=>{'xdspkit'=>{'non_memory_mapped_port'=>'zbt_data_tri'}},'Xilinx'=>{'jtaghwcosim'=>{'non_memory_mapped_port'=>'zbt_data_tri'},'xdspkit'=>{'non_memory_mapped_port'=>'zbt_data_tri'}}}  block_version=VER_STRING_GOES_HERE
  rb1_gw_l_o : xbsIndex_r4/Gateway Out  hdl_port=on  timing_constraint=None  locs_specified=off  LOCs={'A14'}  block_type=gatewayout
      settings: infoedit="Gateway out block.  Converts Xilinx fixed point inputs into ouputs of type Simulink integer, double, or fixed point.<P><P>Hardware notes:  In hardware these blocks become top level output ports or are discarded, depending on how they are configured."  xl_area=[0, 0, 0, 0, 0, 0, 0]  sginterface={'Nallatech'=>{'xdspkit'=>{'non_memory_mapped_port'=>'zbt_rd_wr'}},'Xilinx'=>{'jtaghwcosim'=>{'non_memory_mapped_port'=>'zbt_rd_wr'},'xdspkit'=>{'non_memory_mapped_port'=>'zbt_rd_wr'}}}  block_version=VER_STRING_GOES_HERE
  rb1_q_i : xbsIndex_r4/Gateway In  arith_type=Unsigned  n_bits=10  bin_pt=0  quantization=Truncate  overflow=Wrap  period=(1/fps)/ (rows*(cols+2*blk))  dbl_ovrd=off  timing_constraint=None  locs_specified=off  LOCs={}  block_type=gatewayin
      settings: infoedit="Gateway in block.  Converts inputs of type Simulink integer, double and fixed point to  Xilinx fixed point type.<P><P>Hardware notes:  In hardware these blocks become top level input ports."  xl_area=[0, 0, 0, 0, 0, 0, 0]  sginterface={'Nallatech'=>{'xdspkit'=>{'non_memory_mapped_port'=>'zbt_data_read'}},'Xilinx'=>{'jtaghwcosim'=>{'non_memory_mapped_port'=>'zbt_data_read'},'xdspkit'=>{'non_memory_mapped_port'=>'zbt_data_read'}}}  block_version=VER_STRING_GOES_HERE
  Q : Outport  OutDataType=sfix(16)  OutScaling=2^0
  wires:
  Inverter/1 -> Delay3/1
  Fcn/1 -> Unit Delay3/1
  rb1_gw_l_o/1 -> Fcn/1
  data/1 -> Delay2/1
  rb1_data_tri_o/1 -> Terminator/1
  addr/1 -> rb1_addr_o/1
  we/1 -> Inverter/1
  Unit Delay1/1 -> Unit Delay/1
  rb1_addr_o/1 -> Unit Delay1/1
  Unit Delay3/1 -> Unit Delay2/1
  rb1_q_i/1 -> Q/1
  Unit Delay/1 -> Terminator7/1
  rb1_d_o/1 -> Unit Delay4/1
  Unit Delay2/1 -> Terminator8/1
  Delay2/1 -> rb1_d_o/1
  Unit Delay4/1 -> Unit Delay5/1
  Unit Delay5/1 -> rb1_q_i/1
  Delay3/1 -> rb1_gw_l_o/1, rb1_data_tri_o/1

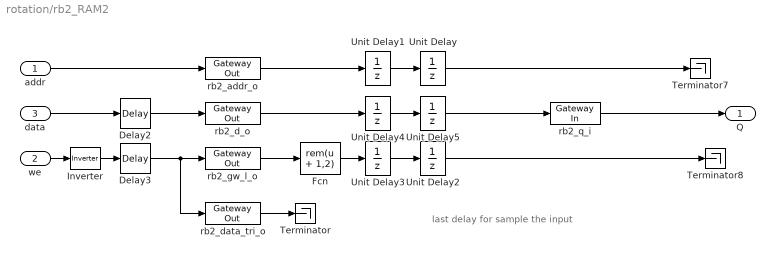
== system rotation/rb2_RAM2 ==
  note: last delay for sample the input
  addr : Inport  OutDataType=sfix(16)  OutScaling=2^0
  we : Inport  Port=2  OutDataType=sfix(16)  OutScaling=2^0
  data : Inport  Port=3  OutDataType=sfix(16)  OutScaling=2^0
  Delay2 : xbsIndex_r4/Delay  en=off  latency=1  dbl_ovrd=off  reg_retiming=off  block_type=delay
      settings: infoedit="Delay line having  configurable length.<P><P>Hardware notes: A delay line is a chain, each link of which is an SRL16 followed by a flip-flop. If register retiming is enabled, the delay line is a chain of flip-flops."  xl_area=[0, 0, 0, 0, 0, 0, 0]  block_version=VER_STRING_GOES_HERE
  Delay3 : xbsIndex_r4/Delay  en=off  latency=1  dbl_ovrd=off  reg_retiming=off  block_type=delay
      settings: infoedit="Delay line having  configurable length.<P><P>Hardware notes: A delay line is a chain, each link of which is an SRL16 followed by a flip-flop. If register retiming is enabled, the delay line is a chain of flip-flops."  xl_area=[0, 0, 0, 0, 0, 0, 0]  block_version=VER_STRING_GOES_HERE
  Fcn : Fcn  Expr=rem(u + 1,2)  SampleTime=(1/fps)/ (rows*(cols+2*blk))
  Inverter : xbsIndex_r4/Inverter  en=off  latency=0  dbl_ovrd=off  block_type=inv
      settings: xl_area=[0, 0, 0, 0, 0, 0, 0]  block_version=VER_STRING_GOES_HERE
  Terminator : Terminator
  Terminator7 : Terminator
  Terminator8 : Terminator
  Unit Delay{,1..5} (6 alike) : UnitDelay  SampleTime=(1/fps)/ (rows*(cols+2*blk))
  rb2_addr_o : xbsIndex_r4/Gateway Out  hdl_port=on  timing_constraint="Data Rate;  Set 'FAST' Attribute"  locs_specified=off  LOCs={'U1','U2','K6','L7','M10','M9','V2','V1','U4','T5','K3','K2','J5','J4','K5','K4','L4','L3'}  block_type=gatewayout
      settings: infoedit="Gateway out block.  Converts Xilinx fixed point inputs into ouputs of type Simulink integer, double, or fixed point.<P><P>Hardware notes:  In hardware these blocks become top level output ports or are discarded, depending on how they are configured."  xl_area=[0, 0, 0, 0, 0, 0, 0]  sginterface={'Nallatech'=>{'xdspkit'=>{'non_memory_mapped_port'=>'zbt_addr'}},'Xilinx'=>{'jtaghwcosim'=>{'non_memory_mapped_port'=>'zbt_addr'},'xdspkit'=>{'non_memory_mapped_port'=>'zbt_addr'}}}  block_version=VER_STRING_GOES_HERE
  rb2_d_o : xbsIndex_r4/Gateway Out  hdl_port=on  timing_constraint=None  locs_specified=off  LOCs={'B21','B22','A22','B23','B19','C19','A20','A21','A23','B24','A24','A25','E18','D18','C18','B18'}  block_type=gatewayout
      settings: infoedit="Gateway out block.  Converts Xilinx fixed point inputs into ouputs of type Simulink integer, double, or fixed point.<P><P>Hardware notes:  In hardware these blocks become top level output ports or are discarded, depending on how they are configured."  xl_area=[0, 0, 0, 0, 0, 0, 0]  sginterface={'Nallatech'=>{'xdspkit'=>{'non_memory_mapped_port'=>'zbt_data'}},'Xilinx'=>{'jtaghwcosim'=>{'non_memory_mapped_port'=>'zbt_data'},'xdspkit'=>{'non_memory_mapped_port'=>'zbt_data'}}}  block_version=VER_STRING_GOES_HERE
  rb2_data_tri_o : xbsIndex_r4/Gateway Out  hdl_port=on  timing_constraint=None  locs_specified=off  LOCs={}  block_type=gatewayout
      settings: infoedit="Gateway out block.  Converts Xilinx fixed point inputs into ouputs of type Simulink integer, double, or fixed point.<P><P>Hardware notes:  In hardware these blocks become top level output ports or are discarded, depending on how they are configured."  xl_area=[0, 0, 0, 0, 0, 0, 0]  sginterface={'Nallatech'=>{'xdspkit'=>{'non_memory_mapped_port'=>'zbt_data_tri'}},'Xilinx'=>{'jtaghwcosim'=>{'non_memory_mapped_port'=>'zbt_data_tri'},'xdspkit'=>{'non_memory_mapped_port'=>'zbt_data_tri'}}}  block_version=VER_STRING_GOES_HERE
  rb2_gw_l_o : xbsIndex_r4/Gateway Out  hdl_port=on  timing_constraint=None  locs_specified=off  LOCs={'A14'}  block_type=gatewayout
      settings: infoedit="Gateway out block.  Converts Xilinx fixed point inputs into ouputs of type Simulink integer, double, or fixed point.<P><P>Hardware notes:  In hardware these blocks become top level output ports or are discarded, depending on how they are configured."  xl_area=[0, 0, 0, 0, 0, 0, 0]  sginterface={'Nallatech'=>{'xdspkit'=>{'non_memory_mapped_port'=>'zbt_rd_wr'}},'Xilinx'=>{'jtaghwcosim'=>{'non_memory_mapped_port'=>'zbt_rd_wr'},'xdspkit'=>{'non_memory_mapped_port'=>'zbt_rd_wr'}}}  block_version=VER_STRING_GOES_HERE
  rb2_q_i : xbsIndex_r4/Gateway In  arith_type=Unsigned  n_bits=10  bin_pt=0  quantization=Truncate  overflow=Wrap  period=(1/fps)/ (rows*(cols+2*blk))  dbl_ovrd=off  timing_constraint=None  locs_specified=off  LOCs={}  block_type=gatewayin
      settings: infoedit="Gateway in block.  Converts inputs of type Simulink integer, double and fixed point to  Xilinx fixed point type.<P><P>Hardware notes:  In hardware these blocks become top level input ports."  xl_area=[0, 0, 0, 0, 0, 0, 0]  sginterface={'Nallatech'=>{'xdspkit'=>{'non_memory_mapped_port'=>'zbt_data_read'}},'Xilinx'=>{'jtaghwcosim'=>{'non_memory_mapped_port'=>'zbt_data_read'},'xdspkit'=>{'non_memory_mapped_port'=>'zbt_data_read'}}}  block_version=VER_STRING_GOES_HERE
  Q : Outport  OutDataType=sfix(16)  OutScaling=2^0
  wires:
  Inverter/1 -> Delay3/1
  Fcn/1 -> Unit Delay3/1
  rb2_gw_l_o/1 -> Fcn/1
  data/1 -> Delay2/1
  rb2_data_tri_o/1 -> Terminator/1
  addr/1 -> rb2_addr_o/1
  we/1 -> Inverter/1
  Unit Delay1/1 -> Unit Delay/1
  rb2_addr_o/1 -> Unit Delay1/1
  Unit Delay3/1 -> Unit Delay2/1
  rb2_q_i/1 -> Q/1
  Unit Delay/1 -> Terminator7/1
  rb2_d_o/1 -> Unit Delay4/1
  Unit Delay2/1 -> Terminator8/1
  Delay2/1 -> rb2_d_o/1
  Unit Delay4/1 -> Unit Delay5/1
  Unit Delay5/1 -> rb2_q_i/1
  Delay3/1 -> rb2_gw_l_o/1, rb2_data_tri_o/1
